simulink model "my_dom_model_2013"  (R2017b)
settings: Solver=VariableStepAuto  StartTime=0.0  StopTime=10000  RelTol=1e-3
undefined symbols (not defined in the file): c_p, C_vp, C_vw, d_f_p, d_T_z, d_T_zew, f_p1, K_1, K_p, K_w, ro_p, steptime, T_p0, T_wew0, T_z1, T_zew1
settings Model: Creator=johnb  LastModifiedBy=johnb

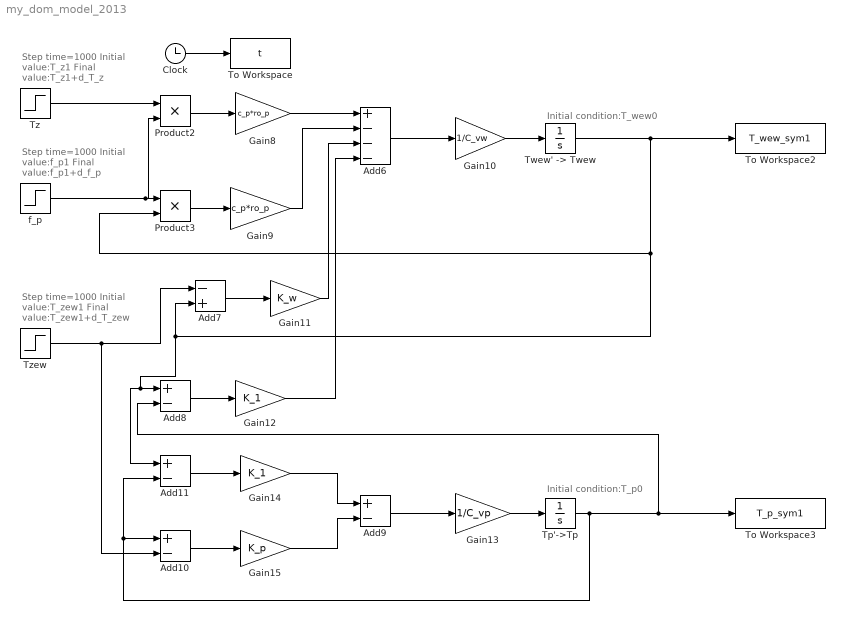
== system my_dom_model_2013 ==
  note: Initial condition:T_p0
  note: Step time=1000
      | Initial value:T_z1
      | Final value:T_z1+d_T_z
  note: Step time=1000
      | Initial value:f_p1
      | Final value:f_p1+d_f_p
  note: Step time=1000
      | Initial value:T_zew1
      | Final value:T_zew1+d_T_zew
  note: Initial condition:T_wew0
  Add{8..11} (4 alike) : Sum  Inputs=+-
  Add6 : Sum  Inputs=+---
  Add7 : Sum  Inputs=-+
  Clock : Clock
  Gain10 : Gain  Gain=1/C_vw
  Gain11 : Gain  Gain=K_w
  Gain12 : Gain  Gain=K_1
  Gain13 : Gain  Gain=1/C_vp
  Gain14 : Gain  Gain=K_1
  Gain15 : Gain  Gain=K_p
  Gain8 : Gain  Gain=c_p*ro_p
  Gain9 : Gain  Gain=c_p*ro_p
  Product2 : Product
  Product3 : Product
  To Workspace : ToWorkspace  VariableName=t  SampleTime=-1
  To Workspace2 : ToWorkspace  VariableName=T_wew_sym1  SampleTime=-1
  To Workspace3 : ToWorkspace  VariableName=T_p_sym1  SampleTime=-1
  Tp'->Tp : Integrator  InitialCondition=T_p0
  "Twew' -> Twew" : Integrator  InitialCondition=T_wew0
  Tz : Step  Time=steptime  Before=T_z1  After=T_z1+d_T_z  SampleTime=0
  "Tzew " : Step  Time=steptime  Before=T_zew1  After=T_zew1+d_T_zew  SampleTime=0
  f_p : Step  Time=steptime  Before=f_p1  After=f_p1+d_f_p  SampleTime=0
  wires:
  Add6/1 -> Gain10/1
  Add11/1 -> Gain14/1
  Add8/1 -> Gain12/1
  Tp'->Tp/1 -> Add8/2, To Workspace3/1, Add11/2, Add10/1
  Add10/1 -> Gain15/1
  Add9/1 -> Gain13/1
  Product3/1 -> Gain9/1
  Gain11/1 -> Add6/3
  Gain10/1 -> "Twew' -> Twew"/1
  Gain15/1 -> Add9/2
  Add7/1 -> Gain11/1
  Gain12/1 -> Add6/4
  Gain14/1 -> Add9/1
  "Tzew "/1 -> Add10/2, Add7/1
  Product2/1 -> Gain8/1
  f_p/1 -> Product2/2, Product3/1
  Gain8/1 -> Add6/1
  Gain9/1 -> Add6/2
  Tz/1 -> Product2/1
  Gain13/1 -> Tp'->Tp/1
  "Twew' -> Twew"/1 -> To Workspace2/1, Product3/2, Add7/2, Add11/1, Add8/1
  Clock/1 -> To Workspace/1
